simulink model "simQ2"  (R2021a)
settings: Solver=VariableStepAuto  StartTime=0.0  StopTime=10  RelTol=1e-3
settings Model: Creator=55189  LastModifiedBy=55189

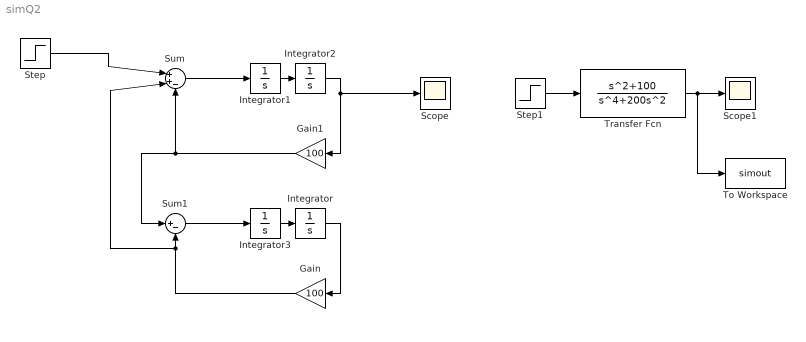
== system simQ2 ==
  Gain : Gain  Gain=100
  Gain1 : Gain  Gain=100
  Integrator{,1..3} (4 alike) : Integrator
  Scope : Scope
  Scope1 : Scope
  Step : Step  Time=0  SampleTime=0
  Step1 : Step  Time=0  SampleTime=0
  Sum : Sum  Inputs=|++-
  Sum1 : Sum  Inputs=|+-
  To Workspace : ToWorkspace  VariableName=simout  SampleTime=-1
  Transfer Fcn : TransferFcn  Numerator=[1 0 100]  Denominator=[1 0 200 0 0]
  wires:
  Sum/1 -> Integrator1/1
  Integrator1/1 -> Integrator2/1
  Integrator2/1 -> Gain1/1, Scope/1
  Step/1 -> Sum/1
  Gain1/1 -> Sum1/1, Sum/3
  Sum1/1 -> Integrator3/1
  Integrator3/1 -> Integrator/1
  Integrator/1 -> Gain/1
  Gain/1 -> Sum/2, Sum1/2
  Transfer Fcn/1 -> To Workspace/1, Scope1/1
  Step1/1 -> Transfer Fcn/1
